simulink model "pilote_automatique"  (R2023a)
settings: Solver=VariableStepAuto  StartTime=0.0  StopTime=t_sim  MinStep=1e-3  RelTol=1e-3
values from neighbouring files (symbols this model uses):
  constantControlInput = 0    [Init_sim.m]
  controlSaturation = 0.5    [Init_sim.m]
  d0 = 10    [Init_sim.m]    (also in suivi_trajectoire.m = 2)
  epsilon = 0    [Init_sim.m]
  gain = 2    [Init_sim.m]
  paramsTrajectoire = [s, a, Omega_0, theta_T0, phi_T0]    [Init_sim.m]
  r = 50    [curve_parametring.m]    (also in parametrage_courbe.m)
  V_WR = 30/3.6    (= 8.33333333333)    [Init_sim.m]
settings Model: Creator=Louis  LastModifiedBy=LouisCassany
settings SolverCC: MaxConsecutiveMinStep=10  ZeroCrossAlgorithm=Adaptive  AlgebraicLoopSolver=TrustRegion
settings DataIOCC: SaveState=on
settings OptimizationCC: ReuseModelBlockBuffer=off
settings DebuggingCC: IgnoredZcDiagnostic=none  UnconnectedInputMsg=warning  UnconnectedOutputMsg=warning  UnconnectedLineMsg=warning  ArithmeticOperatorsInVariantConditions=warning
settings ModelReferenceCC: EnableRefExpFcnMdlSchedulingChecks=on
settings SFSimCC: CustomCodeUndefinedFunction=UseInterfaceOnly

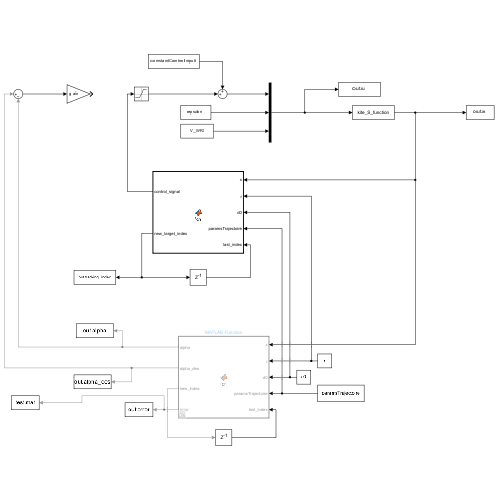
[thumbnail: Simulink's stored preview of the top-level diagram]
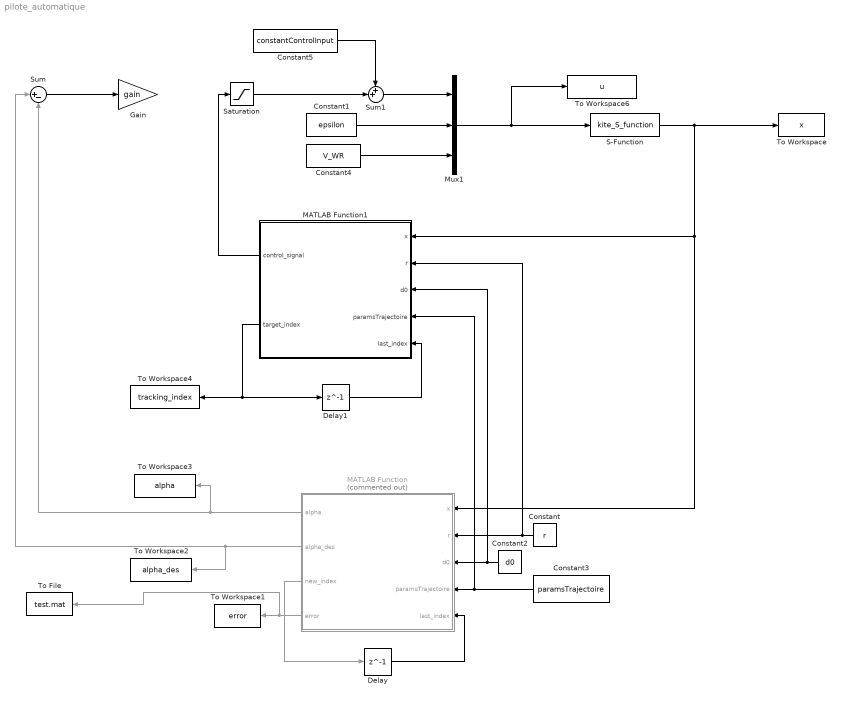
== system pilote_automatique ==
  Constant : Constant  Value=r
  Constant1 : Constant  Value=epsilon
  Constant2 : Constant  Value=d0
  Constant3 : Constant  Value=paramsTrajectoire
  Constant4 : Constant  Value=V_WR
  Constant5 : Constant  Value=constantControlInput
  Delay : Delay  DelayLength=1  InitialCondition=1
  Delay1 : Delay  DelayLength=1  InitialCondition=1
  Gain : Gain  Gain=gain
  MATLAB Function : MATLAB Function  Commented=on  TreatAsAtomicUnit=on
  MATLAB Function1 : MATLAB Function  TreatAsAtomicUnit=on
  Mux1 : Mux  Inputs=3
  S-Function : S-Function  FunctionName=kite_S_function  Parameters=x0  SFunctionDeploymentMode=off  EnableBusSupport=off
  Saturation : Saturate  UpperLimit=controlSaturation  LowerLimit=-controlSaturation
  Sum : Sum  Inputs=|+-
  Sum1 : Sum  Inputs=++|
  To File : ToFile  Filename=test.mat  SaveFormat=Timeseries
  To Workspace : ToWorkspace  VariableName=x  SaveFormat=Timeseries  SampleTime=-1
  To Workspace1 : ToWorkspace  VariableName=error  SaveFormat=Timeseries  SampleTime=-1
  To Workspace2 : ToWorkspace  VariableName=alpha_des  SaveFormat=Timeseries  SampleTime=-1
  To Workspace3 : ToWorkspace  VariableName=alpha  SaveFormat=Timeseries  SampleTime=-1
  To Workspace4 : ToWorkspace  VariableName=tracking_index  SaveFormat=Timeseries  SampleTime=-1
  To Workspace6 : ToWorkspace  VariableName=u  SaveFormat=Timeseries  SampleTime=-1
  wires:
  Constant1/1 -> Mux1/2
  Constant4/1 -> Mux1/3
  Mux1/1 -> To Workspace6/1, S-Function/1
  Constant/1 -> MATLAB Function1/2(r), MATLAB Function/2(r)
  MATLAB Function/3(new_index) -> Delay/1
  Constant2/1 -> MATLAB Function1/3(d0), MATLAB Function/3(d0)
  MATLAB Function/4(error) -> To File/1, To Workspace1/1
  Constant3/1 -> MATLAB Function1/4(paramsTrajectoire), MATLAB Function/4(paramsTrajectoire)
  MATLAB Function/1(alpha) -> To Workspace3/1, Sum/2
  MATLAB Function/2(alpha_des) -> To Workspace2/1, Sum/1
  Sum/1 -> Gain/1
  S-Function/1 -> To Workspace/1, MATLAB Function1/1(x), MATLAB Function/1(x)
  Delay/1 -> MATLAB Function/5(last_index)
  Saturation/1 -> Sum1/2
  Sum1/1 -> Mux1/1
  Constant5/1 -> Sum1/1
  MATLAB Function1/1(control_signal) -> Saturation/1
  Delay1/1 -> MATLAB Function1/5(last_index)
  MATLAB Function1/2(target_index) -> To Workspace4/1, Delay1/1

== matlab function pilote_automatique/MATLAB Function1 ==
  data: x input; control_signal output; r input; d0 input; paramsTrajectoire input; last_index input; target_index output
function [control_signal, target_index]  = fcn(x, r, d0, paramsTrajectoire, last_index)

theta= x(1);
phi = x(2);
psi = x(5);

% phi = 0;
% theta = 50*pi/180;

P = 1;

n = paramsTrajectoire(1);
a = paramsTrajectoire(2);
Omega_T0 = paramsTrajectoire(3);
theta_T0 = paramsTrajectoire(4);
phi_T0 = paramsTrajectoire(5);



[control_signal, alpha, alpha_des, target_index, next_target_index, error] = pilote_auto(theta_T0, phi_T0, n, a, Omega_T0, d0, P, r, last_index, theta, phi, psi);

end

== matlab function pilote_automatique/MATLAB Function ==
  data: x input; alpha output; alpha_des output; r input; d0 input; paramsTrajectoire input; last_index input; new_index output; error output
function [alpha, alpha_des, new_index, error] = fcn(x, r, d0, paramsTrajectoire, last_index)

% persistent Trajectoire;

% if(isempty(Trajectoire))
Trajectoire = get_trajectory(paramsTrajectoire(4),...
    paramsTrajectoire(5),...
    paramsTrajectoire(1),...
    paramsTrajectoire(2),...
    paramsTrajectoire(3));
% end

theta= x(1);
phi = x(2);
psi = x(5);

P_kite = r * [(cos(phi) .* cos(theta)).'; (sin(phi) .* cos(theta)).'; -sin(theta).'];

%% Asservissement en lacet
[alpha1, alpha_des1, new_index1, error1] = asservissement_lacet(P_kite, Trajectoire, d0, last_index, theta, phi, psi);

[alpha, alpha_des, new_index, error2] = pilote_auto(paramsTrajectoire(4),...
    paramsTrajectoire(5),...
    paramsTrajectoire(1),...
    paramsTrajectoire(2),...
    paramsTrajectoire(3),d0, r, last_index, theta, phi, psi);

error = error2 - error1;

end
